simulink model "db_ej_engranes"  (R2018a)
settings: Solver=VariableStepAuto  StartTime=0.0  StopTime=40  RelTol=1e-3
values from neighbouring files (symbols this model uses):
  A = [0 1 ... (first row only)    [ejemplo_engranajes.m]
  A54 = [0 1 ... (first row only)    [ejemplo_engranajes.m]
  B = [0 0 ... (first row only)    [ejemplo_engranajes.m]
  B1 = 450    [ejemplo_engranajes.m]
  B2 = 200    [ejemplo_engranajes.m]
  B54 = [0 0 ... (first row only)    [ejemplo_engranajes.m]
  C = [1 0]    [ejemplo_engranajes.m]
  C54 = [r1/r2 0]    [ejemplo_engranajes.m]
  D = zeros(1,2)    [ejemplo_engranajes.m]
  D54 = zeros(1,2)    [ejemplo_engranajes.m]
  J1 = 0.1    [ejemplo_engranajes.m]
  J2 = 0.5    [ejemplo_engranajes.m]
  K1 = 100    [ejemplo_engranajes.m]
  K2 = 120    [ejemplo_engranajes.m]
  r1 = 0.01    [ejemplo_engranajes.m]
  r2 = 0.05    [ejemplo_engranajes.m]
  u1 = 10    [ejemplo_engranajes.m]
  u2 = 50    [ejemplo_engranajes.m]
settings Model: Creator=carma  LastModifiedBy=carma

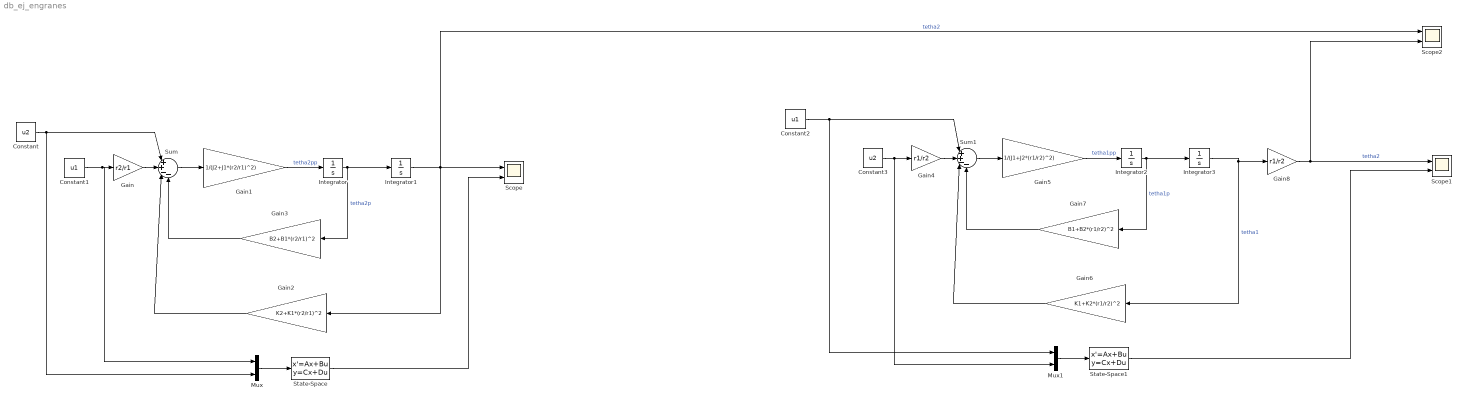
== system db_ej_engranes ==
  Constant : Constant  Value=u2
  Constant1 : Constant  Value=u1
  Constant2 : Constant  Value=u1
  Constant3 : Constant  Value=u2
  Gain : Gain  Gain=r2/r1
  Gain1 : Gain  Gain=1/(J2+J1*(r2/r1)^2)
  Gain2 : Gain  Gain=K2+K1*(r2/r1)^2
  Gain3 : Gain  Gain=B2+B1*(r2/r1)^2
  Gain4 : Gain  Gain=r1/r2
  Gain5 : Gain  Gain=1/(J1+J2*(r1/r2)^2)
  Gain6 : Gain  Gain=K1+K2*(r1/r2)^2
  Gain7 : Gain  Gain=B1+B2*(r1/r2)^2
  Gain8 : Gain  Gain=r1/r2
  Integrator{,1..3} (4 alike) : Integrator
  Mux : Mux  Inputs=2
  Mux1 : Mux  Inputs=2
  Scope : Scope  NumInputPorts=2
  Scope1 : Scope  NumInputPorts=2
  Scope2 : Scope  NumInputPorts=2
  State-Space : StateSpace  A=A  B=B  C=C  D=D  InitialCondition=0
  State-Space1 : StateSpace  A=A54  B=B54  C=C54  D=D54  InitialCondition=0
  Sum : Sum  Inputs=|++--
  Sum1 : Sum  Inputs=|++--
  wires:
  Constant/1 -> Mux/2, Sum/1
  Gain/1 -> Sum/2
  Constant1/1 -> Mux/1, Gain/1
  Sum/1 -> Gain1/1
  Gain1/1 -> Integrator/1  "tetha2pp"
  Integrator/1 -> Gain3/1, Integrator1/1  "tetha2p"
  Integrator1/1 -> Scope2/1, Gain2/1, Scope/1  "tetha2"
  Gain2/1 -> Sum/3
  Gain3/1 -> Sum/4
  Mux/1 -> State-Space/1
  State-Space/1 -> Scope/2
  State-Space1/1 -> Scope1/2
  Mux1/1 -> State-Space1/1
  Gain5/1 -> Integrator2/1  "tetha1pp"
  Sum1/1 -> Gain5/1
  Integrator2/1 -> Gain7/1, Integrator3/1  "tetha1p"
  Integrator3/1 -> Gain6/1, Gain8/1  "tetha1"
  Constant2/1 -> Mux1/1, Sum1/1
  Gain7/1 -> Sum1/4
  Gain4/1 -> Sum1/2
  Constant3/1 -> Mux1/2, Gain4/1
  Gain6/1 -> Sum1/3
  Gain8/1 -> Scope2/2, Scope1/1  "tetha2"
